simulink model "pid1kgk"  (R2020b)
settings: Solver=VariableStepAuto  StartTime=0.0  StopTime=10  RelTol=1e-3
libraries: pid_lib x3
settings Model: Creator=lamth  LastModifiedBy=lamth

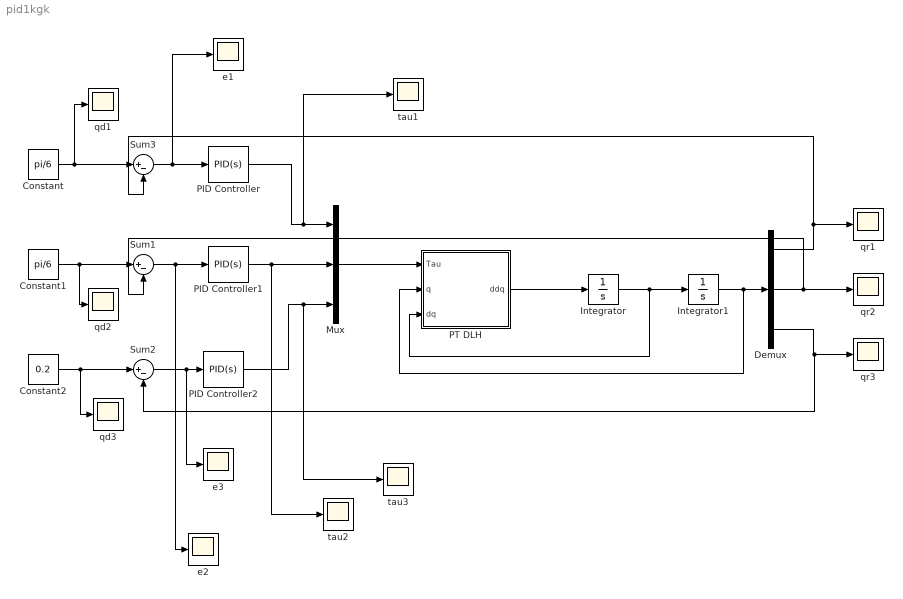
== system pid1kgk ==
  Constant : Constant  Value=pi/6
  Constant1 : Constant  Value=pi/6
  Constant2 : Constant  Value=0.2
  Demux : Demux  Outputs=3
  Integrator : Integrator
  Integrator1 : Integrator
  Mux : Mux  Inputs=3
  PID Controller : pid_lib/PID Controller  Controller=PID  Form=Parallel  TimeDomain=Continuous-time  UseExternalTs=off  SampleTime=-1  IntegratorMethod=Forward Euler  FilterMethod=Forward Euler  ControllerParametersSource=internal  P=380.929228733311  I=363.866326757805  D=94.529010644806  UseFilter=on  N=47.9435324134581  TunerSelectOption=Transfer Function Based (PID Tuner App)  InitialConditionSource=internal  InitialConditionForIntegrator=0  InitialConditionForFilter=0  DifferentiatorICPrevScaledInput=0  ExternalReset=none  TrackingMode=off  Kt=1  LimitOutput=off  SatLimitsSource=internal  UpperSaturationLimit=inf  LowerSaturationLimit=-inf  LinearizeAsGain=on  AntiWindupMode=none  Kb=1  POutMin=[]  POutMax=[]  IOutMin=[]  IOutMax=[]  DOutMin=[]  DOutMax=[]  NOutMin=[]  NOutMax=[]  SumOutMin=[]  SumOutMax=[]  SaturationOutMin=[]  SaturationOutMax=[]  PParamMin=[]  PParamMax=[]  IParamMin=[]  IParamMax=[]  DParamMin=[]  DParamMax=[]  NParamMin=[]  NParamMax=[]  KbParamMin=[]  KbParamMax=[]  KtParamMin=[]  KtParamMax=[]  KbOutMin=[]  KbOutMax=[]  KtOutMin=[]  KtOutMax=[]  IntegratorOutMin=[]  IntegratorOutMax=[]  FilterOutMin=[]  FilterOutMax=[]  SumI1OutMin=[]  SumI1OutMax=[]  SumI2OutMin=[]  SumI2OutMax=[]  SumI3OutMin=[]  SumI3OutMax=[]  SumI4OutMin=[]  SumI4OutMax=[]  SumDOutMin=[]  SumDOutMax=[]  DifferentiatorOutMin=[]  DifferentiatorOutMax=[]  FilterDiffOutCoefMin=[]  FilterDiffOutCoefMax=[]  ReciprocalOutMin=[]  ReciprocalOutMax=[]  SumDenOutMin=[]  SumDenOutMax=[]  SumNumOutMin=[]  SumNumOutMax=[]  DivideOutMin=[]  DivideOutMax=[]  UdiffTsProdOutMin=[]  UdiffTsProdOutMax=[]  NTsProdOutMin=[]  NTsProdOutMax=[]  UintegralTsProdOutMin=[]  UintegralTsProdOutMax=[]  UngainTsProdOutMin=[]  UngainTsProdOutMax=[]  IntegratorContinuousStateAttributes=''  IntegratorStateMustResolveToSignalObject=off  IntegratorRTWStateStorageClass=Auto  FilterContinuousStateAttributes=''  FilterStateMustResolveToSignalObject=off  FilterRTWStateStorageClass=Auto  ParallelPVariant=InternalParameters  IdealPVariant=Disabled  IVariant=InternalParameters  DVariant=InternalParameters  IntegratorVariant=Continuous  SatVariant=Disabled  AWVariant=Passthrough  PCopyVariant=Disabled  TRVariant=Disabled  FdbkBlocksVariant=Forward  IdealPFdbkVariant=Disabled  SatFdbkVariant=Disabled  DerivativeFilterVariant=ContFilter  NVariant=InternalParameters  NCopyVariant=Disabled  FilterICVariant=InternalICsFilter  IntegratorICVariant=InternalICs  ExternalResetVariant=Disabled  TRSumVariant=Passthrough  SumFdbkVariant=Disabled  SumVariant=Sum_PID  TsampFilterVariant=InternalTs  TsampNgainVariant=Passthrough  TsampIntegralVariant=Passthrough  ExternalSaturationOutDataTypeStr=Inherit: Same as second input
  PID Controller1 : pid_lib/PID Controller  Controller=PID  Form=Parallel  TimeDomain=Continuous-time  UseExternalTs=off  SampleTime=-1  IntegratorMethod=Forward Euler  FilterMethod=Forward Euler  ControllerParametersSource=internal  P=337.232938444831  I=155.368202244432  D=15.5120993248899  UseFilter=on  N=6150.42854499099  TunerSelectOption=Transfer Function Based (PID Tuner App)  InitialConditionSource=internal  InitialConditionForIntegrator=0  InitialConditionForFilter=0  DifferentiatorICPrevScaledInput=0  ExternalReset=none  TrackingMode=off  Kt=1  LimitOutput=off  SatLimitsSource=internal  UpperSaturationLimit=inf  LowerSaturationLimit=-inf  LinearizeAsGain=on  AntiWindupMode=none  Kb=1  POutMin=[]  POutMax=[]  IOutMin=[]  IOutMax=[]  DOutMin=[]  DOutMax=[]  NOutMin=[]  NOutMax=[]  SumOutMin=[]  SumOutMax=[]  SaturationOutMin=[]  SaturationOutMax=[]  PParamMin=[]  PParamMax=[]  IParamMin=[]  IParamMax=[]  DParamMin=[]  DParamMax=[]  NParamMin=[]  NParamMax=[]  KbParamMin=[]  KbParamMax=[]  KtParamMin=[]  KtParamMax=[]  KbOutMin=[]  KbOutMax=[]  KtOutMin=[]  KtOutMax=[]  IntegratorOutMin=[]  IntegratorOutMax=[]  FilterOutMin=[]  FilterOutMax=[]  SumI1OutMin=[]  SumI1OutMax=[]  SumI2OutMin=[]  SumI2OutMax=[]  SumI3OutMin=[]  SumI3OutMax=[]  SumI4OutMin=[]  SumI4OutMax=[]  SumDOutMin=[]  SumDOutMax=[]  DifferentiatorOutMin=[]  DifferentiatorOutMax=[]  FilterDiffOutCoefMin=[]  FilterDiffOutCoefMax=[]  ReciprocalOutMin=[]  ReciprocalOutMax=[]  SumDenOutMin=[]  SumDenOutMax=[]  SumNumOutMin=[]  SumNumOutMax=[]  DivideOutMin=[]  DivideOutMax=[]  UdiffTsProdOutMin=[]  UdiffTsProdOutMax=[]  NTsProdOutMin=[]  NTsProdOutMax=[]  UintegralTsProdOutMin=[]  UintegralTsProdOutMax=[]  UngainTsProdOutMin=[]  UngainTsProdOutMax=[]  IntegratorContinuousStateAttributes=''  IntegratorStateMustResolveToSignalObject=off  IntegratorRTWStateStorageClass=Auto  FilterContinuousStateAttributes=''  FilterStateMustResolveToSignalObject=off  FilterRTWStateStorageClass=Auto  ParallelPVariant=InternalParameters  IdealPVariant=Disabled  IVariant=InternalParameters  DVariant=InternalParameters  IntegratorVariant=Continuous  SatVariant=Disabled  AWVariant=Passthrough  PCopyVariant=Disabled  TRVariant=Disabled  FdbkBlocksVariant=Forward  IdealPFdbkVariant=Disabled  SatFdbkVariant=Disabled  DerivativeFilterVariant=ContFilter  NVariant=InternalParameters  NCopyVariant=Disabled  FilterICVariant=InternalICsFilter  IntegratorICVariant=InternalICs  ExternalResetVariant=Disabled  TRSumVariant=Passthrough  SumFdbkVariant=Disabled  SumVariant=Sum_PID  TsampFilterVariant=InternalTs  TsampNgainVariant=Passthrough  TsampIntegralVariant=Passthrough  ExternalSaturationOutDataTypeStr=Inherit: Same as second input
  PID Controller2 : pid_lib/PID Controller  Controller=PID  Form=Parallel  TimeDomain=Continuous-time  UseExternalTs=off  SampleTime=-1  IntegratorMethod=Forward Euler  FilterMethod=Forward Euler  ControllerParametersSource=internal  P=50  I=30  D=20  UseFilter=on  N=100  TunerSelectOption=Transfer Function Based (PID Tuner App)  InitialConditionSource=internal  InitialConditionForIntegrator=0  InitialConditionForFilter=0  DifferentiatorICPrevScaledInput=0  ExternalReset=none  TrackingMode=off  Kt=1  LimitOutput=off  SatLimitsSource=internal  UpperSaturationLimit=inf  LowerSaturationLimit=-inf  LinearizeAsGain=on  AntiWindupMode=none  Kb=1  POutMin=[]  POutMax=[]  IOutMin=[]  IOutMax=[]  DOutMin=[]  DOutMax=[]  NOutMin=[]  NOutMax=[]  SumOutMin=[]  SumOutMax=[]  SaturationOutMin=[]  SaturationOutMax=[]  PParamMin=[]  PParamMax=[]  IParamMin=[]  IParamMax=[]  DParamMin=[]  DParamMax=[]  NParamMin=[]  NParamMax=[]  KbParamMin=[]  KbParamMax=[]  KtParamMin=[]  KtParamMax=[]  KbOutMin=[]  KbOutMax=[]  KtOutMin=[]  KtOutMax=[]  IntegratorOutMin=[]  IntegratorOutMax=[]  FilterOutMin=[]  FilterOutMax=[]  SumI1OutMin=[]  SumI1OutMax=[]  SumI2OutMin=[]  SumI2OutMax=[]  SumI3OutMin=[]  SumI3OutMax=[]  SumI4OutMin=[]  SumI4OutMax=[]  SumDOutMin=[]  SumDOutMax=[]  DifferentiatorOutMin=[]  DifferentiatorOutMax=[]  FilterDiffOutCoefMin=[]  FilterDiffOutCoefMax=[]  ReciprocalOutMin=[]  ReciprocalOutMax=[]  SumDenOutMin=[]  SumDenOutMax=[]  SumNumOutMin=[]  SumNumOutMax=[]  DivideOutMin=[]  DivideOutMax=[]  UdiffTsProdOutMin=[]  UdiffTsProdOutMax=[]  NTsProdOutMin=[]  NTsProdOutMax=[]  UintegralTsProdOutMin=[]  UintegralTsProdOutMax=[]  UngainTsProdOutMin=[]  UngainTsProdOutMax=[]  IntegratorContinuousStateAttributes=''  IntegratorStateMustResolveToSignalObject=off  IntegratorRTWStateStorageClass=Auto  FilterContinuousStateAttributes=''  FilterStateMustResolveToSignalObject=off  FilterRTWStateStorageClass=Auto  ParallelPVariant=InternalParameters  IdealPVariant=Disabled  IVariant=InternalParameters  DVariant=InternalParameters  IntegratorVariant=Continuous  SatVariant=Disabled  AWVariant=Passthrough  PCopyVariant=Disabled  TRVariant=Disabled  FdbkBlocksVariant=Forward  IdealPFdbkVariant=Disabled  SatFdbkVariant=Disabled  DerivativeFilterVariant=ContFilter  NVariant=InternalParameters  NCopyVariant=Disabled  FilterICVariant=InternalICsFilter  IntegratorICVariant=InternalICs  ExternalResetVariant=Disabled  TRSumVariant=Passthrough  SumFdbkVariant=Disabled  SumVariant=Sum_PID  TsampFilterVariant=InternalTs  TsampNgainVariant=Passthrough  TsampIntegralVariant=Passthrough  ExternalSaturationOutDataTypeStr=Inherit: Same as second input
  PT DLH : MATLAB Function  TreatAsAtomicUnit=on
  Sum1 : Sum  Inputs=|+-
  Sum2 : Sum  Inputs=|+-
  Sum3 : Sum  Inputs=|+-
  e1 : Scope
  e2 : Scope
  e3 : Scope
  qd1 : Scope
  qd2 : Scope
  qd3 : Scope
  qr1 : Scope
  qr2 : Scope
  qr3 : Scope
  tau1 : Scope
  tau2 : Scope
  tau3 : Scope
  wires:
  Constant1/1 -> qd2/1, Sum1/1
  Constant2/1 -> qd3/1, Sum2/1
  Constant/1 -> qd1/1, Sum3/1
  PT DLH/1(ddq) -> Integrator/1
  Integrator/1 -> PT DLH/3(dq), Integrator1/1
  Sum3/1 -> e1/1, PID Controller/1
  Sum1/1 -> PID Controller1/1, e2/1
  Sum2/1 -> e3/1, PID Controller2/1
  Mux/1 -> PT DLH/1(Tau)
  Integrator1/1 -> PT DLH/2(q), Demux/1
  Demux/2 -> qr2/1, Sum1/2
  Demux/1 -> Sum3/2, qr1/1
  Demux/3 -> Sum2/2, qr3/1
  PID Controller1/1 -> tau2/1, Mux/2
  PID Controller/1 -> tau1/1, Mux/1
  PID Controller2/1 -> tau3/1, Mux/3

== matlab function pid1kgk/PT DLH ==
  data: Tau input; q input; ddq output; dq input
function ddq  = fcn(Tau,q,dq)
[m1,m2,m3,L1,L2,L3,I1x,I1y,I1z,I2x,I2y,I2z,I3x,I3y,I3z]=parameter ();

q=zeros(3,1);
dq=zeros(3,1);

% Khai bao ma tran khoi luong M
M=zeros(3,3);
M(1,1)= (9/4)*m1*L1^2+I1z+3*m2*L2*L1*cos(q(2))+L1^2*m2+(9/4)*m2*L2^2+I2y+2*m3*L2*L1*cos(q(2))+3*m3*L1*q(3)*sin(q(2))+L1^2*m3+L2^2*m3+(9/4)*m3*q(3)^2+I3y;
M(1,2)= (3/2)*m2*L2*L1*cos(q(2))+(9/4)*m2*L2^2+I2y+m3*L2*L1*cos(q(2))+(3/2)*m3*L1*q(3)*sin(q(2))+L2^2*m3+(9/4)*m3*q(3)^2+I3y;
M(1,3)= -(3/2)*L1*m3*cos(q(2))-(3/2)*L2*m3;


M(2,1)=(3/2)*m2*L2*L1*cos(q(2))+(9/4)*m2*L2^2+I2y+m3*L2*L1*cos(q(2))+(3/2)*m3*L1*q(3)*sin(q(2))+L2^2*m3+(9/4)*m3*q(3)^2+I3y;
M(2,2)=(9/4)*m2*L2^2+I2y+L2^2*m3+(9/4)*m3*q(3)^2+I3y;
M(2,3)=-(3/2)*L2*m3;

M(3,1)=-(3/2)*L1*m3*cos(q(2))-(3/2)*L2*m3;
M(3,2)=-(3/2)*L2*m3;
M(3,3)=(9/4)*m3;

% Khai bao ma tran Coriolis C
%h=-m2*L1*Lc2*sin(q(2));
Co=zeros(3,3);
Co(1,1)=-3*L1*L2*sin(q(2))*dq(2)*m2-2*L1*L2*sin(q(2))*dq(2)*m3+3*L1*cos(q(2))*dq(2)*m3*q(3)+3*L1*m3*sin(q(2))*dq(3)+(9/2)*m3*q(3)*dq(3);
Co(1,2)=-(3/2)*L1*L2*sin(q(2))*dq(2)*m2-L1*L2*sin(q(2))*dq(2)*m3+(3/2)*L1*cos(q(2))*dq(2)*m3*q(3)+(3/2)*L1*m3*sin(q(2))*dq(3)+(9/2)*m3*q(3)*dq(3);
Co(1,3)=(3/2)*L1*m3*sin(q(2))*dq(2);


Co(2,1)=(3/2)*L1*L2*sin(q(2))*dq(1)*m2+L1*L2*sin(q(2))*dq(1)*m3-(3/4)*L1*L2*sin(q(2))*dq(2)*m2-(1/2)*L1*L2*sin(q(2))*dq(2)*m3-(3/2)*L1*cos(q(2))*dq(1)*m3*q(3)+(3/4)*L1*cos(q(2))*dq(2)*m3*q(3)+(3/4)*L1*m3*sin(q(2))*dq(3)+(9/2)*m3*q(3)*dq(3);
Co(2,2)=(3/4)*L1*L2*sin(q(2))*dq(1)*m2+(1/2)*L1*L2*sin(q(2))*dq(1)*m3-(3/4)*L1*cos(q(2))*dq(1)*m3*q(3)+(9/2)*m3*q(3)*dq(3);
Co(2,3)=-(3/4)*L1*m3*sin(q(2))*dq(1);


Co(3,1)=-(3/2)*L1*m3*sin(q(2))*dq(1)+(3/4)*L1*m3*sin(q(2))*dq(2)-(9/4)*dq(1)*m3*q(3)-(9/4)*m3*q(3)*dq(2);
Co(3,2)=-(3/4)*L1*m3*sin(q(2))*dq(1)-(9/4)*dq(1)*m3*q(3)-(9/4)*m3*q(3)*dq(2);
Co(3,3)=0;

% Ma tran the nang hap dan
G=zeros(3,1);
G(1,1)=15*m1*L1*cos(q(1))+10*m2*L1*cos(q(1))+10*m3*L1*cos(q(1))+15*m2*L2*cos(q(1)+q(2))+10*m3*L2*cos(q(1)+q(2))+15*m3*sin(q(1)+q(2))*q(3);
G(2,1)=15*m2*L2*cos(q(1)+q(2))+10*m3*L2*cos(q(1)+q(2))+15*m3*sin(q(1)+q(2))*q(3);
G(3,1)=-15*m3*cos(q(1)+q(2));


% Pt DLH
ddq=inv(M)*(Tau-Co*dq-G);
